simulink model "sampleModel1720_1_sub_sub"  (R2023a)
settings: Solver=VariableStepAuto  StartTime=0.0  StopTime=10.0  RelTol=1e-3
libraries: hdlsllib x4
settings Model: Creator=user1  LastModifiedBy=user1

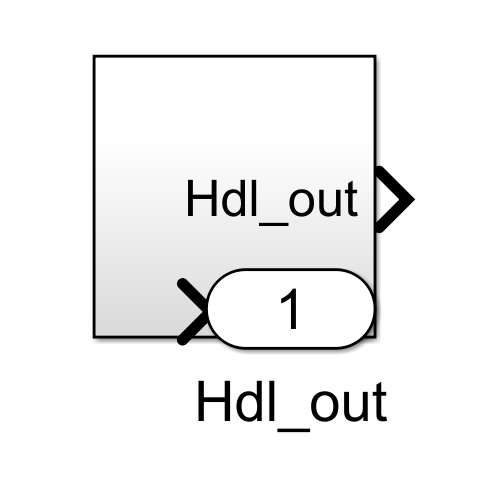
[thumbnail: Simulink's stored preview of the top-level diagram]
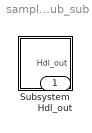
== system sampleModel1720_1_sub_sub ==
  Subsystem : Subsystem
  Hdl_out : Outport  OutDataTypeStr=uint8

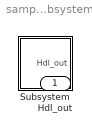
== system sampleModel1720_1_sub_sub/Subsystem ==
  Subsystem : Subsystem
  Hdl_out : Outport  OutDataTypeStr=uint8

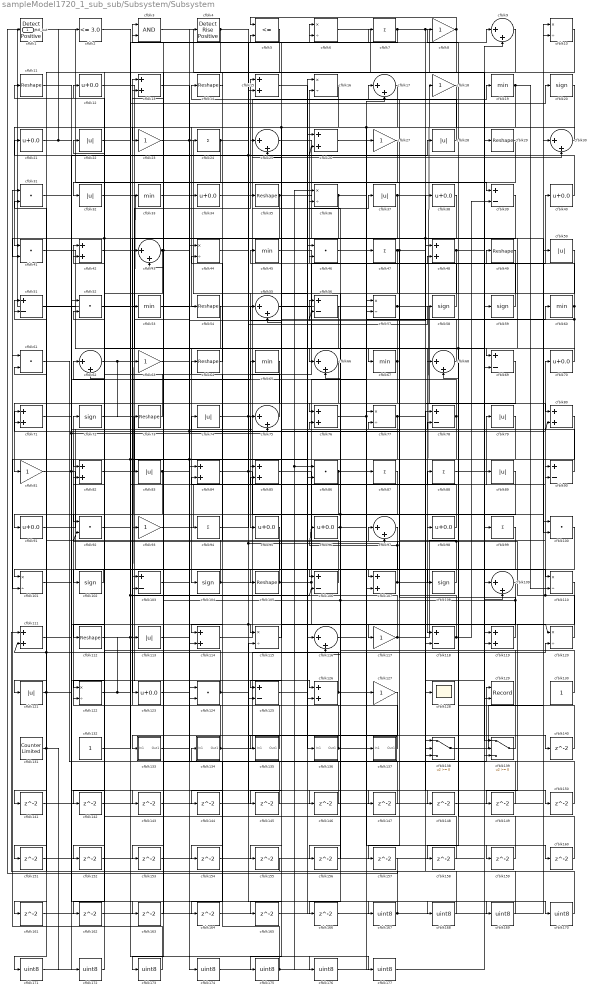
== system sampleModel1720_1_sub_sub/Subsystem/Subsystem ==
  cfblk1 : hdlsllib/Logic and Bit Operations/Detect Rise Positive  vinit=0  OutDataTypeStr=uint8
  cfblk{6,10,16,36,44,57,77,101,110,115,120,122} (12 alike) : Product  Inputs=*/  OutDataTypeStr=uint8  RndMeth=Zero  SaturateOnIntegerOverflow=on
  cfblk{31,41,46,52,61,86,92,100,124} (9 alike) : DotProduct  OutDataTypeStr=uint8
  cfblk{20,58..59,72,102,104,108} (7 alike) : Signum
  cfblk{39,51,56,69,78,90,103,106,118,125} (10 alike) : Sum  Inputs=+-  OutDataTypeStr=uint8
  cfblk{11,14,29,35,49,54,64,73,105,112} (10 alike) : Reshape
  cfblk{13,15,26,42,48,71,76,80,82,84..85,107,111,114,119,126} (16 alike) : Sum  OutDataTypeStr=uint8
  cfblk{9,17,25,30,43,55,62,66,68,75,97,109,116} (13 alike) : Sum  Inputs=|++  OutDataTypeStr=uint8
  cfblk{22,28,32,37,50,74,79,83,89,113,121} (11 alike) : Abs  OutDataTypeStr=uint8  SaturateOnIntegerOverflow=off
  cfblk{8,18,23,27,63,81,93,117,127} (9 alike) : Gain  OutDataTypeStr=uint8
  cfblk{12,21,34,38,40,70,91,95..96,98,123} (11 alike) : Bias  Bias=0.0  SaturateOnIntegerOverflow=off
  cfblk128 : Scope
  cfblk129 : Record  FileSettingsInternal="{\"entries\":[{\"content\":{\"excelSettings\":{\"content\":{},\"type\":\"Streamout.ExcelSettings\"}},\"type\":\"Streamout.FileSettingStorage\",\"uuid\":\"\"}],\"packageUris\":[\"http:\\/\\/schema.mathworks.com\\/mf0\\/streamout_blocks\\/R2020a\"],\"version\":\"1.0\"}"  Layout=[1 1]  SignalsInternal="{\"entries\":[{\"content\":{\"signals\":[{\"content\":{\"blockPath\":[],\"dimensions\":[1],\"domain\":\"\",\"lineColor\":\"#a2142f\",\"plots\":[1],\"port\":1,\"signalID\":36914,\"signalName\":\"cfblk61\"},\"type\":\"RecordBlkView.Signal\",\"uuid\":\"\"},{\"content\":{\"blockPath\":[],\"dimensions\":[1],\"domain\":\"\",\"lineColor\":\"#139fff\",\"plots\":[1],\"port\":2,\"signalID\":36917,\"signalName\":\"cfblk7\"},\"type\":\"RecordBlkView.Signal\",\"uuid\":\"\"}]},\"type\":\"RecordBlkView.InputSignals\",\"uuid\":\"\"}],\"packageUris\":[\"http:\\/\\/schema.mathworks.com\\/mf0\\/streamout_blocks\\/R2020a\"],\"version\":\"1.0\"}"  VisualizationBindings="{\"xyplotplugin\":{\"info\":[{\"series\":[{\"bindingParametersList\":[{\"parameter\":\"X-Axis\",\"signalID\":36914,\"signalName\":\"cfblk61\"},{\"parameter\":\"Y-Axis\",\"signalID\":36917,\"signalName\":\"cfblk7\"}],\"seriesID\":22147}],\"subplotID\":1}]}}"  CompatibilityTag=XY  st=-1
  cfblk130 : Constant  OutDataTypeStr=uint8  SampleTime=-1
  cfblk131 : hdlsllib/Sources/Counter Limited  uplimit=7  tsamp=-1
  cfblk132 : Constant  OutDataTypeStr=uint8  SampleTime=-1
  cfblk133 : Subsystem
      settings: LibrarySourceBlock=|
      | hdlsllib/Ports &
      | Subsystems/Subsystem
  cfblk134 : Subsystem
      settings: LibrarySourceBlock=|
      | hdlsllib/Ports &
      | Subsystems/Subsystem
  cfblk135 : Subsystem
      settings: LibrarySourceBlock=|
      | hdlsllib/Ports &
      | Subsystems/Subsystem
  cfblk136 : Subsystem
      settings: LibrarySourceBlock=|
      | hdlsllib/Ports &
      | Subsystems/Subsystem
  cfblk137 : Subsystem
      settings: LibrarySourceBlock=|
      | hdlsllib/Ports &
      | Subsystems/Subsystem
  cfblk138 : Switch  OutDataTypeStr=uint8  SaturateOnIntegerOverflow=off  InputSameDT=off
  cfblk139 : Switch  OutDataTypeStr=uint8  SaturateOnIntegerOverflow=off  InputSameDT=off
  cfblk{140..166} (27 alike) : Delay  SampleTime=1
  cfblk{167..177} (11 alike) : DataTypeConversion  OutDataTypeStr=uint8  SaturateOnIntegerOverflow=off  RndMeth=Floor
  cfblk{19,33,45,53,60,65,67} (7 alike) : MinMax  OutDataTypeStr=uint8
  cfblk2 : hdlsllib/Logic and Bit Operations/Compare To Constant  relop=<=  const=3.0  OutDataTypeStr=uint8
  cfblk{7,24,47,87..88,94,99} (7 alike) : Sum  Inputs=+  OutDataTypeStr=uint8
  cfblk3 : Logic  AllPortsSameDT=off  OutDataTypeStr=boolean
  cfblk4 : hdlsllib/Logic and Bit Operations/Detect Rise Positive  vinit=0  OutDataTypeStr=uint8
  cfblk5 : RelationalOperator  Operator=<=  OutDataTypeStr=boolean  InputSameDT=off
  Hdl_out : Outport  OutDataTypeStr=uint8
  wires:
  cfblk177/1 -> cfblk109/2
  cfblk63/1 -> cfblk177/1
  cfblk176/1 -> cfblk109/1
  cfblk175/1 -> cfblk36/1, cfblk86/1, cfblk134/1(In1)
  cfblk174/1 -> cfblk127/1
  cfblk103/1 -> cfblk174/1
  cfblk173/1 -> cfblk61/1
  cfblk127/1 -> cfblk173/1
  cfblk172/1 -> cfblk52/2
  cfblk171/1 -> cfblk52/1
  cfblk9/1 -> cfblk171/1
  cfblk170/1 -> cfblk78/1
  cfblk52/1 -> cfblk170/1
  cfblk169/1 -> cfblk31/2
  cfblk168/1 -> cfblk31/1
  cfblk167/1 -> cfblk50/1, cfblk42/2
  cfblk166/1 -> cfblk10/2
  cfblk165/1 -> cfblk126/2
  cfblk164/1 -> cfblk46/1
  cfblk5/1 -> cfblk164/1
  cfblk163/1 -> cfblk3/2
  cfblk11/1 -> cfblk163/1
  cfblk162/1 -> cfblk62/1
  cfblk65/1 -> cfblk162/1
  cfblk161/1 -> cfblk17/2
  cfblk160/1 -> cfblk68/2
  cfblk159/1 -> cfblk139/2
  cfblk158/1 -> cfblk122/2
  cfblk157/1 -> cfblk1/1
  cfblk50/1 -> cfblk157/1
  cfblk156/1 -> cfblk66/2
  cfblk80/1 -> cfblk156/1
  cfblk155/1 -> cfblk111/1
  cfblk56/1 -> cfblk155/1
  cfblk154/1 -> cfblk107/2
  cfblk38/1 -> cfblk154/1
  cfblk153/1 -> cfblk139/3
  cfblk152/1 -> cfblk16/1
  cfblk151/1 -> cfblk138/3
  cfblk150/1 -> cfblk138/2
  cfblk149/1 -> cfblk84/1
  cfblk110/1 -> cfblk149/1
  cfblk148/1 -> cfblk48/2
  cfblk26/1 -> cfblk148/1
  cfblk147/1 -> cfblk116/2
  cfblk146/1 -> cfblk13/2
  cfblk92/1 -> cfblk146/1
  cfblk145/1 -> cfblk124/1
  cfblk97/1 -> cfblk145/1
  cfblk144/1 -> cfblk9/2
  cfblk143/1 -> cfblk118/2
  cfblk142/1 -> cfblk30/1
  cfblk87/1 -> cfblk142/1
  cfblk141/1 -> cfblk115/2
  cfblk69/1 -> cfblk141/1
  cfblk140/1 -> cfblk78/2
  cfblk37/1 -> cfblk114/2, cfblk100/2
  cfblk124/1 -> cfblk12/1, cfblk140/1
  cfblk109/1 -> cfblk175/1
  cfblk86/1 -> cfblk135/1(In1), cfblk160/1
  cfblk78/1 -> cfblk124/2, cfblk101/2, cfblk63/1
  cfblk46/1 -> cfblk47/1
  cfblk89/1 -> cfblk106/1, cfblk144/1
  cfblk101/1 -> cfblk74/1
  cfblk20/1 -> cfblk55/2
  cfblk133/1(Out1) -> cfblk4/1
  cfblk123/1 -> cfblk56/1, cfblk80/2
  cfblk108/1 -> cfblk92/2, cfblk71/2
  cfblk106/1 -> cfblk64/1
  cfblk64/1 -> cfblk44/2
  cfblk134/1(Out1) -> cfblk120/2, cfblk93/1
  cfblk53/1 -> cfblk35/1
  cfblk132/1 -> cfblk20/1
  cfblk25/1 -> cfblk108/1
  cfblk22/1 -> cfblk7/1
  cfblk136/1(Out1) -> cfblk87/1, cfblk22/1
  cfblk34/1 -> cfblk30/2
  cfblk67/1 -> cfblk3/1, cfblk166/1
  cfblk51/1 -> cfblk119/2
  cfblk68/1 -> cfblk21/1
  cfblk76/1 -> cfblk60/1, cfblk159/1
  cfblk15/1 -> cfblk68/1
  cfblk139/1 -> cfblk46/2
  cfblk60/1 -> cfblk82/1, cfblk158/1, cfblk56/2, cfblk25/2
  cfblk14/1 -> cfblk114/1
  cfblk126/1 -> cfblk111/2, cfblk51/1, cfblk90/2
  cfblk18/1 -> cfblk41/1
  cfblk120/1 -> cfblk97/1, cfblk90/1
  cfblk44/1 -> cfblk120/1, cfblk147/1, cfblk97/2
  cfblk94/1 -> cfblk15/2
  cfblk88/1 -> cfblk29/1
  cfblk6/1 -> cfblk119/1
  cfblk100/1 -> cfblk103/1
  cfblk1/1 -> cfblk137/1(In1)
  cfblk57/1 -> cfblk89/1, Hdl_out/1
  cfblk116/1 -> cfblk88/1
  cfblk115/1 -> cfblk45/1
  cfblk79/1 -> cfblk121/1
  cfblk138/1 -> cfblk10/1
  cfblk39/1 -> cfblk92/1, cfblk41/2
  cfblk81/1 -> cfblk136/1(In1), cfblk125/2
  cfblk29/1 -> cfblk62/2
  cfblk10/1 -> cfblk34/1
  cfblk77/1 -> cfblk150/1, cfblk151/1
  cfblk19/1 -> cfblk57/2, cfblk125/1, cfblk110/2
  cfblk31/1 -> cfblk167/1
  cfblk49/1 -> cfblk69/2
  cfblk40/1 -> cfblk25/1
  cfblk102/1 -> cfblk101/1
  cfblk82/1 -> cfblk44/1
  cfblk105/1 -> cfblk27/1, cfblk139/1, cfblk82/2
  cfblk16/1 -> cfblk105/1, cfblk94/1
  cfblk113/1 -> cfblk24/1
  cfblk84/1 -> cfblk26/2, cfblk6/1, cfblk138/1
  cfblk21/1 -> cfblk2/1, cfblk143/1
  cfblk59/1 -> cfblk8/1
  cfblk24/1 -> cfblk43/1, cfblk39/1
  cfblk130/1 -> cfblk71/1
  cfblk91/1 -> cfblk38/1
  cfblk42/1 -> cfblk53/1
  cfblk90/1 -> cfblk55/1
  cfblk96/1 -> cfblk57/1, cfblk76/2
  cfblk30/1 -> cfblk23/1
  cfblk83/1 -> cfblk91/1, cfblk168/1
  cfblk62/1 -> cfblk15/1, cfblk73/1
  cfblk8/1 -> cfblk133/1(In1), cfblk5/1
  cfblk99/1 -> cfblk118/1
  cfblk13/1 -> cfblk85/1
  cfblk131/1 -> cfblk61/2, cfblk172/1
  cfblk55/1 -> cfblk40/1
  cfblk66/1 -> cfblk81/1
  cfblk3/1 -> cfblk48/1
  cfblk2/1 -> cfblk86/2, cfblk176/1
  cfblk23/1 -> cfblk95/1, cfblk6/2
  cfblk112/1 -> cfblk33/1, cfblk85/2
  cfblk27/1 -> cfblk32/1
  cfblk47/1 -> cfblk117/1, cfblk80/1, cfblk76/1
  cfblk125/1 -> cfblk26/1
  cfblk33/1 -> cfblk116/1
  cfblk98/1 -> cfblk84/2
  cfblk45/1 -> cfblk98/1
  cfblk122/1 -> cfblk9/1, cfblk106/2, cfblk113/1
  cfblk17/1 -> cfblk54/1
  cfblk35/1 -> cfblk128/1, cfblk100/1, cfblk123/1
  cfblk119/1 -> cfblk43/2, cfblk36/2, cfblk77/2
  cfblk135/1(Out1) -> cfblk13/1
  cfblk121/1 -> cfblk65/1, cfblk75/2, cfblk161/1
  cfblk93/1 -> cfblk79/1
  cfblk70/1 -> cfblk66/1
  cfblk73/1 -> cfblk11/1
  cfblk111/1 -> cfblk115/1
  cfblk41/1 -> cfblk104/1
  cfblk118/1 -> cfblk17/1, cfblk39/2
  cfblk12/1 -> cfblk67/1
  cfblk104/1 -> cfblk19/1, cfblk51/2
  cfblk95/1 -> cfblk122/1
  cfblk36/1 -> cfblk77/1, cfblk83/1
  cfblk7/1 -> cfblk59/1, cfblk129/2, cfblk5/2
  cfblk4/1 -> cfblk112/1, cfblk169/1
  cfblk75/1 -> cfblk42/1
  cfblk71/1 -> cfblk28/1
  cfblk58/1 -> cfblk16/2
  cfblk43/1 -> cfblk110/1, cfblk153/1, cfblk152/1
  cfblk107/1 -> cfblk75/1, cfblk96/1, cfblk18/1
  cfblk117/1 -> cfblk70/1, cfblk103/2
  cfblk74/1 -> cfblk37/1, cfblk58/1
  cfblk48/1 -> cfblk99/1, cfblk165/1
  cfblk61/1 -> cfblk129/1
  cfblk32/1 -> cfblk69/1
  cfblk114/1 -> cfblk49/1
  cfblk54/1 -> cfblk102/1
  cfblk85/1 -> cfblk107/1
  cfblk137/1(Out1) -> cfblk72/1
  cfblk72/1 -> cfblk126/1
  cfblk28/1 -> cfblk14/1

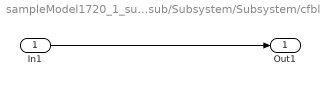
== system sampleModel1720_1_sub_sub/Subsystem/Subsystem/cfblk133 ==
  In1 : Inport
  Out1 : Outport
  wires:
  In1/1 -> Out1/1

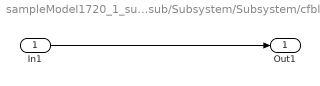
== system sampleModel1720_1_sub_sub/Subsystem/Subsystem/cfblk134 ==
  In1 : Inport
  Out1 : Outport
  wires:
  In1/1 -> Out1/1

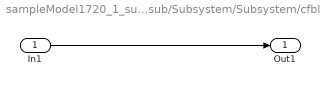
== system sampleModel1720_1_sub_sub/Subsystem/Subsystem/cfblk135 ==
  In1 : Inport
  Out1 : Outport
  wires:
  In1/1 -> Out1/1

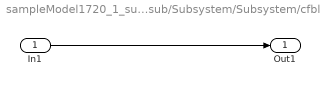
== system sampleModel1720_1_sub_sub/Subsystem/Subsystem/cfblk136 ==
  In1 : Inport
  Out1 : Outport
  wires:
  In1/1 -> Out1/1

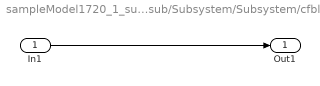
== system sampleModel1720_1_sub_sub/Subsystem/Subsystem/cfblk137 ==
  In1 : Inport
  Out1 : Outport
  wires:
  In1/1 -> Out1/1
